simulink model "GalvoTransferFunc"  (Simulink 8.1)
settings: Solver=ode45  StartTime=0.0  StopTime=0.05  FixedStep=0.000005  MaxStep=5e-4  MinStep=5e-6  RelTol=1e-3
libraries: simulink x2
settings Model: Creator=mainster  LastModifiedBy=mainster  BufferReuse=off
settings OptimizationCC: OptimizeBlockIOStorage=off  BufferReuse=off  ExpressionFolding=off  LocalBlockOutputs=off

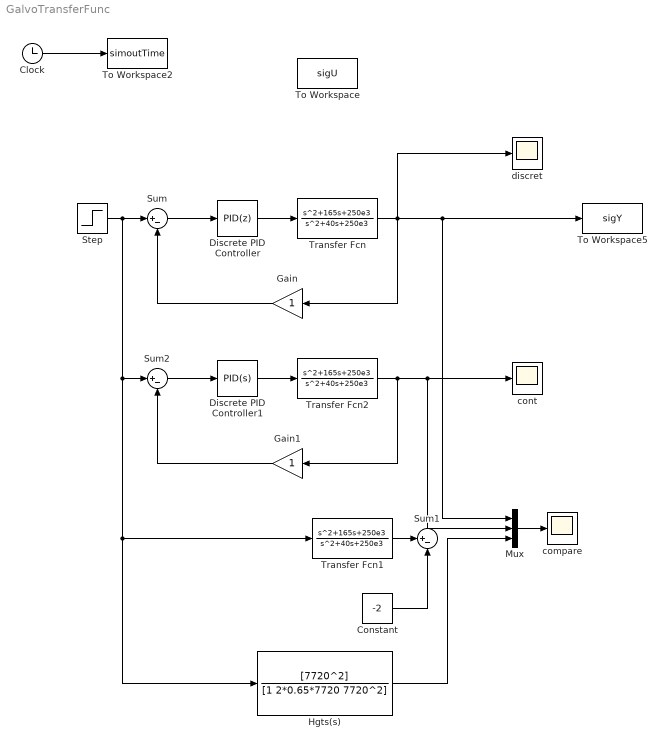
== system GalvoTransferFunc ==
  Clock : Clock
  Constant : Constant  Value=-2
  Discrete PID Controller : simulink/Continuous/PID Controller  Controller=PID  TimeDomain=Discrete-time  SampleTime=100e-6  IntegratorMethod=Forward Euler  FilterMethod=Forward Euler  Form=Parallel  P=0.476188758625585  I=9523.77517251169  D=0  N=100  InitialConditionSource=internal  InitialConditionForIntegrator=0  InitialConditionForFilter=0  ExternalReset=none  LimitOutput=off  UpperSaturationLimit=inf  LowerSaturationLimit=-inf  LinearizeAsGain=off  AntiWindupMode=none  Kb=1  TrackingMode=off  Kt=1  PParamMin=[]  PParamMax=[]  IParamMin=[]  IParamMax=[]  DParamMin=[]  DParamMax=[]  NParamMin=[]  NParamMax=[]  KbParamMin=[]  KbParamMax=[]  KtParamMin=[]  KtParamMax=[]  POutMin=[]  POutMax=[]  IOutMin=[]  IOutMax=[]  DOutMin=[]  DOutMax=[]  NOutMin=[]  NOutMax=[]  KbOutMin=[]  KbOutMax=[]  KtOutMin=[]  KtOutMax=[]  IntegratorOutMin=[]  IntegratorOutMax=[]  FilterOutMin=[]  FilterOutMax=[]  SumOutMin=[]  SumOutMax=[]  SumI1OutMin=[]  SumI1OutMax=[]  SumI2OutMin=[]  SumI2OutMax=[]  SumI3OutMin=[]  SumI3OutMax=[]  SumDOutMin=[]  SumDOutMax=[]  SaturationOutMin=[]  SaturationOutMax=[]  IntegratorContinuousStateAttributes=''  IntegratorStateMustResolveToSignalObject=off  IntegratorRTWStateStorageClass=Auto  FilterContinuousStateAttributes=''  FilterStateMustResolveToSignalObject=off  FilterRTWStateStorageClass=Auto
  Discrete PID Controller1 : simulink/Continuous/PID Controller  Controller=PID  TimeDomain=Continuous-time  SampleTime=100e-6  IntegratorMethod=Forward Euler  FilterMethod=Forward Euler  Form=Parallel  P=0  I=1825.87590895877  D=0  N=100  InitialConditionSource=internal  InitialConditionForIntegrator=0  InitialConditionForFilter=0  ExternalReset=none  LimitOutput=off  UpperSaturationLimit=inf  LowerSaturationLimit=-inf  LinearizeAsGain=off  AntiWindupMode=none  Kb=1  TrackingMode=off  Kt=1  PParamMin=[]  PParamMax=[]  IParamMin=[]  IParamMax=[]  DParamMin=[]  DParamMax=[]  NParamMin=[]  NParamMax=[]  KbParamMin=[]  KbParamMax=[]  KtParamMin=[]  KtParamMax=[]  POutMin=[]  POutMax=[]  IOutMin=[]  IOutMax=[]  DOutMin=[]  DOutMax=[]  NOutMin=[]  NOutMax=[]  KbOutMin=[]  KbOutMax=[]  KtOutMin=[]  KtOutMax=[]  IntegratorOutMin=[]  IntegratorOutMax=[]  FilterOutMin=[]  FilterOutMax=[]  SumOutMin=[]  SumOutMax=[]  SumI1OutMin=[]  SumI1OutMax=[]  SumI2OutMin=[]  SumI2OutMax=[]  SumI3OutMin=[]  SumI3OutMax=[]  SumDOutMin=[]  SumDOutMax=[]  SaturationOutMin=[]  SaturationOutMax=[]  IntegratorContinuousStateAttributes=''  IntegratorStateMustResolveToSignalObject=off  IntegratorRTWStateStorageClass=Auto  FilterContinuousStateAttributes=''  FilterStateMustResolveToSignalObject=off  FilterRTWStateStorageClass=Auto
  Gain : Gain
  Gain1 : Gain
  Hgts(s) : TransferFcn  Numerator=[7720^2]  Denominator=[1 2*0.65*7720 7720^2]
  Mux : Mux  Inputs=3
  Step : Step  Time=0.01  SampleTime=0
  Sum : Sum  Inputs=|+-
  Sum1 : Sum  Inputs=|+-
  Sum2 : Sum  Inputs=|+-
  To Workspace : ToWorkspace  VariableName=sigU  SampleTime=-1  SaveFormat=Structure
  To Workspace2 : ToWorkspace  VariableName=simoutTime  SampleTime=-1  SaveFormat=Structure
  To Workspace5 : ToWorkspace  VariableName=sigY  SampleTime=-1  SaveFormat=Structure
  Transfer Fcn : TransferFcn  Numerator=[1 165 250e3]  Denominator=[1 40 250e3]
  Transfer Fcn1 : TransferFcn  Numerator=[1 165 250e3]  Denominator=[1 40 250e3]
  Transfer Fcn2 : TransferFcn  Numerator=[1 165 250e3]  Denominator=[1 40 250e3]
  compare : Scope
      settings: TickLabels=on  ShowLegends=on  TimeRange=0.05  YMin=0  YMax=1.4  SaveName=ScopeData2
  cont : Scope
  discret : Scope
  wires:
  Clock/1 -> To Workspace2/1
  Step/1 -> Sum/1, Sum2/1, Transfer Fcn1/1, Hgts(s)/1
  Sum/1 -> Discrete PID Controller/1
  Transfer Fcn/1 -> Gain/1, discret/1, To Workspace5/1, Mux/1
  Discrete PID Controller/1 -> Transfer Fcn/1
  Gain/1 -> Sum/2
  Transfer Fcn1/1 -> Sum1/1
  Constant/1 -> Sum1/2
  Sum2/1 -> Discrete PID Controller1/1
  Transfer Fcn2/1 -> Gain1/1, cont/1, Mux/2
  Discrete PID Controller1/1 -> Transfer Fcn2/1
  Gain1/1 -> Sum2/2
  Mux/1 -> compare/1
  Hgts(s)/1 -> Mux/3
